simulink model "P5_6_MassSpringDamping"  (R2025b)
settings: Solver=VariableStepAuto  StartTime=0.0  StopTime=100  MaxStep=1e-2  RelTol=1e-3
settings Model: Creator=tongx  LastModifiedBy=tongx

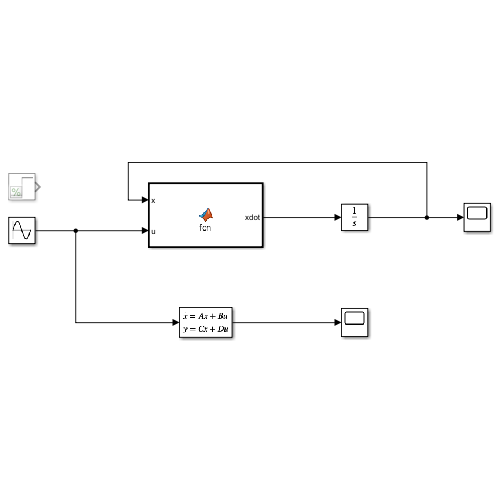
[thumbnail: Simulink's stored preview of the top-level diagram]
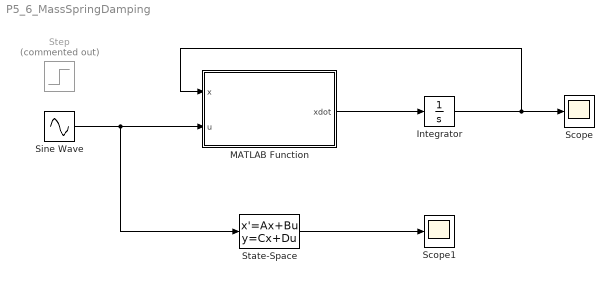
== system P5_6_MassSpringDamping ==
  Integrator : Integrator  InitialCondition=[1 0].'
  MATLAB Function : MATLAB Function  TreatAsAtomicUnit=on
  Scope : Scope
      settings: ActiveDisplayYMinimum=-6.2496163464122407  ActiveDisplayYMaximum=6.2496019879851969
  Scope1 : Scope
      settings: ActiveDisplayYMinimum=-6.2494935026333316  ActiveDisplayYMaximum=6.2495883386764293
  Sine Wave : Sin  SampleTime=0
  State-Space : StateSpace  A=[0 1; -1 -0.2];  B=[0 1]';  C=[1 0]  D=0  InitialCondition=[1 0].'
  Step : Step  Commented=on  SampleTime=0
  wires:
  MATLAB Function/1(xdot) -> Integrator/1
  Integrator/1 -> Scope/1, MATLAB Function/1(x)
  Sine Wave/1 -> State-Space/1, MATLAB Function/2(u)
  State-Space/1 -> Scope1/1

== matlab function P5_6_MassSpringDamping/MATLAB Function ==
  data: x input; u input; xdot output
function xdot = fcn(x, u)

m = 1;
k = 1;
b = 0.2;

xdot = [x(2)
    -k/m*x(1)-b/m*x(2)+u/m];
